simulink library "SG_library"  (R2020a)
settings: Solver=VariableStepAuto  StartTime=0.0  StopTime=10.0  RelTol=1e-3
undefined symbols (not defined in the file): a, b, c, IO334, IO334_IO_FPGA, IO334_IO_src, IO334_SOS_FPGA, IO334_SOS_src, IO397, IO397_IO_FPGA, IO397_IO_src, IO397_SOS_FPGA, IO397_SOS_src
libraries: speedgoatlib_hdlCoder_IO3xx x35, $bdroot x20, xpcutilitieslib x8, hdlsllib x5, simulink x4, simulink_extras x1
(part 1 of 2)
settings Model: Creator=mavolery  LastModifiedBy=mavolery
settings SFSimCC: CustomCodeUndefinedFunction=UseInterfaceOnly

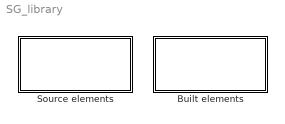
== system SG_library ==
  Built elements : Subsystem
  Source elements : Subsystem

== system SG_library/Built elements ==
  IO334_IO : Subsystem  mask(IO334 IO){ts=20e-6, OutputRange=Auto (same as ADC)}
      mask prompts: ts "Sampling time"; OutputRange "DAC Voltage Range:"
      mask help: Links the 16 first physical analog inputs/outputs to the CPU part of the speedgoat.
      mask TypeOptions OutputRange: IO334_IO_FPGA/OutputRange
      mask DialogControl AnalogOutput Prompt: Analog Output
  IO334_SOS : Subsystem  mask(IO334_SOS){sos1=[0 0 0 1 0 0;0 0 0 1 0 0;0 0 0 1 0 0;0 0 0 1 0 0], sos2=[0 0 0 1 0 0;0 0 0 1 0 0;0 0 0 1 0 0;0 0 0 1 0 0], limit_ctrl=10, ts=20e-6, os=1}
      mask prompts: sos1 "SOS matrix AI1 -> AO1"; sos2 "SOS matrix AI2 -> AO1"; limit_ctrl "Control output limit [V]"; ts "Sampling time (ADC)"; os "Oversampling (f_adc/f_cpu)"
      mask help: Implements a discrete fixed-point filter by second order sections cascade. SOS matrices are given by tf2sos or zp2sos.
  IO397_IO : Subsystem  mask(IO397 IO){ts=50e-6, range1=+-5 V, range2=+-5.12 V, range3=+-10 V, range4=+-10.24 V, span=+-10 V}
      mask prompts: ts "Sampling time:"; range1 "Range ADC Channel 1"; range2 "Range ADC Channel 2"; range3 "Range ADC Channel 3"; range4 "Range ADC Channel 4"; span "DAC Voltage Span:"
      mask help: Links the four first physical analog inputs/outputs to the CPU part of the speedgoat.
      mask TypeOptions range1: IO397_IO_FPGA/range1
      mask TypeOptions range2: IO397_IO_FPGA/range2
      mask TypeOptions range3: IO397_IO_FPGA/range3
      mask TypeOptions range4: IO397_IO_FPGA/range4
      mask TypeOptions span: IO397_IO_FPGA/span
      mask DialogControl AnalogInput Prompt: Analog Inputs
      mask DialogControl AnalogOutput Prompt: Analog Output
  IO397_SOS : Subsystem  mask(IO397_SOS){sos1=[1 0 0 1 0 0;1 0 0 1 0 0;1 0 0 1 0 0;1 0 0 1 0 0], sos2=[0 0 0 1 0 0;0 0 0 1 0 0;0 0 0 1 0 0;0 0 0 1 0 0], limit_ctrl=10, ts=50e-6, os=1, range1=+-10 V, range2=+-10 V, range3=+-10 V, range4=+-10 V, span=+-10 V}
      mask prompts: sos1 "SOS matrix AI1 -> AO1"; sos2 "SOS matrix AI2 -> AO1"; limit_ctrl "Control output limit [V]"; ts "Sampling time (ADC)"; os "Oversampling (f_adc/f_cpu)"; range1 "Range ADC Channel 1"; range2 "Range ADC Channel 2"; range3 "Range ADC Channel 3"; range4 "Range ADC Channel 4"; span "DAC Voltage Span:"
      mask help: Implements a discrete fixed-point filter by second order sections cascade. SOS matrices are given by tf2sos or zp2sos.
      mask init:
      | assert(all(range1 ~= [1 4 5]), 'ADC1 range must be symetric');
      | assert(all(range2 ~= [1 4 5]), 'ADC2 range must be symetric');
      | assert(all(span ~= [1 2]), 'DAC span must be symetric');
      mask TypeOptions range1: IO397_SOS_FPGA/range1
      mask TypeOptions range2: IO397_SOS_FPGA/range2
      mask TypeOptions range3: IO397_SOS_FPGA/range3
      mask TypeOptions range4: IO397_SOS_FPGA/range4
      mask TypeOptions span: IO397_SOS_FPGA/span
      mask DialogControl AnalogInput Prompt: Analog Inputs
      mask DialogControl AnalogOutput Prompt: Analog Output
  private : Subsystem

== system SG_library/Source elements ==
  ADC trigger : Subsystem  mask(AI trigger){}
      mask help: Creates a boolean pulse every given cylces. It can be use for ADC acquisition
  Discrete SOS section DFII serial : Subsystem  mask(Discrete fixed-point SOS section){idx=1}
      mask prompts: idx "Index"
      mask help:
      | This is a fixed-point implementation of a biquad filter. Specify the sos [N/2, 6] matrix e.g. given by tf2sos or zpk2sos functions. The first denominator coefficient must always be equal to 1. Index (1 - N/2) parameter specifies which section of the filter is implemented.
      |
      | This is the same implementation as in LabView VI "Discrete Transfer Function Direct.vi" or order 2. It has same fixed-point implementation too.
  Discrete SOS serial : Subsystem  mask(Discrete fixed-point second order sections filter){}
      mask help: This is a SOS implemetation of order 8 (4 sections). Specify the sos [n/2, 6] matrix e.g. given by tf2sos function. The first denominator coefficient must always be equal to 1.
  IO334 DAC double2fi : Subsystem  mask(DAC double2fi){span=1}
      mask help:
      | Converts the double signal to the fi(1,16,15) value for feeding the FPGA
      | Span is defined as follows:
      | 1 -> 0V - 5V
      | 2 -> 0V - 10V
      | 3 -> -5V - 5V
      | 4 -> -10V - 10V
  IO397 ADC fi2double : Subsystem  mask(ADC fi2double){range=1}
      mask help:
      | Converts the fi(1,16,15) signal from the FPGA to a double value
      | Range is defined as follows:
      | 1 -> 0V - 5.12V
      | 2 -> 0V - 10V (acts as -5V - 5V on IO397)
      | 3 -> 0V - 10.24V (acts as -5.12V - 5.12V on IO397)
      | 4 -> -5V - 5V (acts as 0V - 10V on IO397)
      | 5 -> -5.12V - 5.12V (acts as 0V - 10.24V on IO397)
      | 6 -> -10V - 10V
      | 7 -> -10.24V - 10.24V
  IO397 DAC double2fi : Subsystem  mask(DAC double2fi){span=1}
      mask help:
      | Converts the double signal to the fi(1,16,15) value for feeding the FPGA
      | Span is defined as follows:
      | 1 -> 0V - 5V
      | 2 -> 0V - 10V
      | 3 -> -5V - 5V
      | 4 -> -10V - 10V
  Random source : Subsystem  mask(Random source){mean=0, stdev=1, seed=0, SampleTime=0.0001}
      mask prompts: stdev "Standard deviation"; SampleTime "Sample time"
      mask help: Creates some random signal, limited in frequency at Fs/4
  Saturation : Subsystem  mask(Saturation){}
      mask help: Saturates the signal between -limit and limit.
  Triggered Pulse : Subsystem  mask(Triggered Pulse){}
      mask help: Generates a single pulse of N samples length

== system SG_library/Built elements/IO334_IO ==
  note: ADC range is not tuneable
  AO : Inport
  Data Type Conversion3 : DataTypeConversion  OutDataTypeStr=double
  Gain4 : Gain  Gain=20
  Ground : Ground
  IO334 DAC double2fi1 : $bdroot/Source elements/IO334 DAC double2fi  span=OutputRange
  IO334_IO_FPGA : $bdroot/Built elements/private/IO334_IO_FPGA  module_id=1  slot=-1  ts=-1  OutputRange=Auto (same as ADC)  FpgaFreq=100
  Mux : Mux  Inputs=26
  Rate Transition : RateTransition  OutPortSampleTime=ts
  Terminator : Terminator
  AI : Outport  VectorParamsAs1DForOutWhenUnconnected=off
  wires:
  AO/1 -> Rate Transition/1
  Data Type Conversion3/1 -> Gain4/1
  Gain4/1 -> AI/1
  IO334_IO_FPGA/27 -> Data Type Conversion3/1
  Rate Transition/1 -> IO334 DAC double2fi1/1
  IO334 DAC double2fi1/1 -> IO334_IO_FPGA/25
  Ground/1 -> IO334_IO_FPGA/1, IO334_IO_FPGA/2, IO334_IO_FPGA/3, IO334_IO_FPGA/4, IO334_IO_FPGA/5, IO334_IO_FPGA/6, IO334_IO_FPGA/7, IO334_IO_FPGA/8, IO334_IO_FPGA/9, IO334_IO_FPGA/10, IO334_IO_FPGA/11, IO334_IO_FPGA/12, IO334_IO_FPGA/13, IO334_IO_FPGA/14, IO334_IO_FPGA/15, IO334_IO_FPGA/16, IO334_IO_FPGA/17, IO334_IO_FPGA/18, IO334_IO_FPGA/19, IO334_IO_FPGA/20, IO334_IO_FPGA/21, IO334_IO_FPGA/22, IO334_IO_FPGA/23, IO334_IO_FPGA/24
  IO334_IO_FPGA/1 -> Mux/1
  IO334_IO_FPGA/2 -> Mux/2
  IO334_IO_FPGA/3 -> Mux/3
  IO334_IO_FPGA/4 -> Mux/4
  IO334_IO_FPGA/5 -> Mux/5
  IO334_IO_FPGA/6 -> Mux/6
  IO334_IO_FPGA/7 -> Mux/7
  IO334_IO_FPGA/8 -> Mux/8
  IO334_IO_FPGA/9 -> Mux/9
  IO334_IO_FPGA/10 -> Mux/10
  IO334_IO_FPGA/11 -> Mux/11
  IO334_IO_FPGA/12 -> Mux/12
  IO334_IO_FPGA/13 -> Mux/13
  IO334_IO_FPGA/14 -> Mux/14
  IO334_IO_FPGA/15 -> Mux/15
  IO334_IO_FPGA/16 -> Mux/16
  IO334_IO_FPGA/17 -> Mux/17
  IO334_IO_FPGA/18 -> Mux/18
  IO334_IO_FPGA/19 -> Mux/19
  IO334_IO_FPGA/20 -> Mux/20
  IO334_IO_FPGA/21 -> Mux/21
  IO334_IO_FPGA/22 -> Mux/22
  IO334_IO_FPGA/23 -> Mux/23
  IO334_IO_FPGA/24 -> Mux/24
  IO334_IO_FPGA/25 -> Mux/25
  IO334_IO_FPGA/26 -> Mux/26
  Mux/1 -> Terminator/1

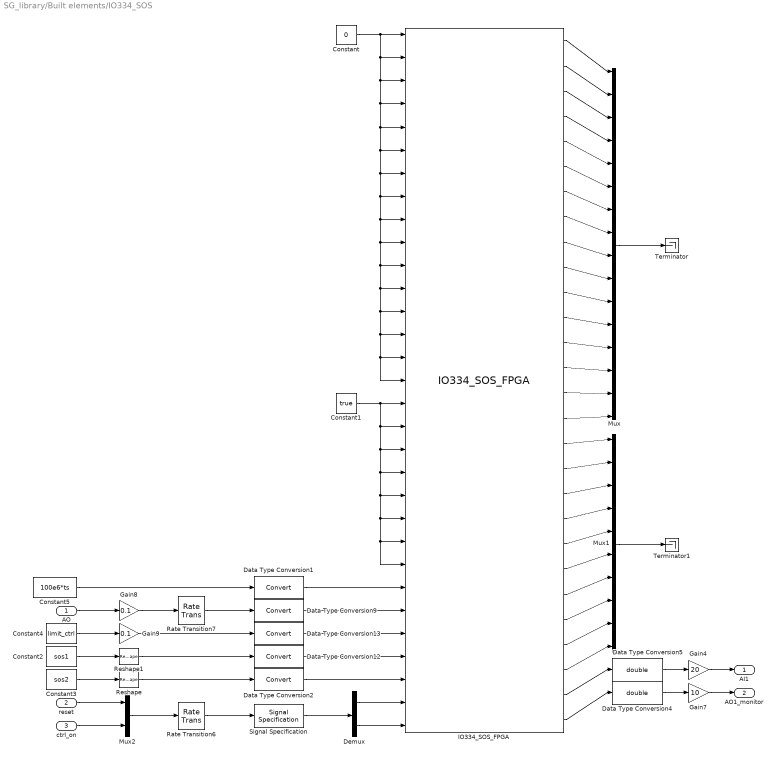
== system SG_library/Built elements/IO334_SOS ==
  AO : Inport
  reset : Inport  Port=2
  ctrl_on : Inport  Port=3
  Constant : Constant  Value=0  OutDataTypeStr=Inherit: Inherit via back propagation  SampleTime=-1
  Constant1 : Constant  Value=true  OutDataTypeStr=Inherit: Inherit via back propagation  SampleTime=-1
  Constant2 : Constant  Value=sos1  SampleTime=-1
  Constant3 : Constant  Value=sos2  SampleTime=-1
  Constant4 : Constant  Value=limit_ctrl  SampleTime=-1
  Constant5 : Constant  Value=100e6*ts  SampleTime=-1
  Data Type Conversion{1..2,9,12} (4 alike) : DataTypeConversion  RndMeth=Simplest
  Data Type Conversion13 : DataTypeConversion  RndMeth=Simplest  SaturateOnIntegerOverflow=on
  Data Type Conversion4 : DataTypeConversion  OutDataTypeStr=double
  Data Type Conversion5 : DataTypeConversion  OutDataTypeStr=double
  Demux : Demux  Outputs=2
  Gain4 : Gain  Gain=20
  Gain7 : Gain  Gain=10
  Gain8 : Gain  Gain=0.1
  Gain9 : Gain  Gain=0.1
  IO334_SOS_FPGA : $bdroot/Built elements/private/IO334_SOS_FPGA  module_id=1  slot=-1  ts=-1  OutputRange=Auto (same as ADC)  FpgaFreq=100
  Mux : Mux  Inputs=16
  Mux1 : Mux  Inputs=10
  Mux2 : Mux  Inputs=2
  Rate Transition6 : RateTransition
  Rate Transition7 : RateTransition  OutPortSampleTime=ts*os
  Reshape : Reshape
  Reshape1 : Reshape
  Signal Specification : SignalSpecification  OutDataTypeStr=boolean
  Terminator : Terminator
  Terminator1 : Terminator
  AI1 : Outport  VectorParamsAs1DForOutWhenUnconnected=off
  AO1_monitor : Outport  Port=2  VectorParamsAs1DForOutWhenUnconnected=off
  wires:
  Data Type Conversion5/1 -> Gain4/1
  Rate Transition6/1 -> Signal Specification/1
  Data Type Conversion4/1 -> Gain7/1
  Gain4/1 -> AI1/1
  Gain7/1 -> AO1_monitor/1
  Constant4/1 -> Gain9/1
  Gain9/1 -> Data Type Conversion13/1
  Signal Specification/1 -> Demux/1
  Constant2/1 -> Reshape1/1
  Constant3/1 -> Reshape/1
  Rate Transition7/1 -> Data Type Conversion9/1
  Gain8/1 -> Rate Transition7/1
  AO/1 -> Gain8/1
  Constant5/1 -> Data Type Conversion1/1
  Data Type Conversion1/1 -> IO334_SOS_FPGA/25
  Data Type Conversion9/1 -> IO334_SOS_FPGA/26
  Data Type Conversion13/1 -> IO334_SOS_FPGA/27
  Demux/2 -> IO334_SOS_FPGA/31
  Demux/1 -> IO334_SOS_FPGA/30
  Mux2/1 -> Rate Transition6/1
  ctrl_on/1 -> Mux2/2
  reset/1 -> Mux2/1
  Constant1/1 -> IO334_SOS_FPGA/17, IO334_SOS_FPGA/18, IO334_SOS_FPGA/19, IO334_SOS_FPGA/20, IO334_SOS_FPGA/21, IO334_SOS_FPGA/22, IO334_SOS_FPGA/23, IO334_SOS_FPGA/24
  Constant/1 -> IO334_SOS_FPGA/1, IO334_SOS_FPGA/2, IO334_SOS_FPGA/3, IO334_SOS_FPGA/4, IO334_SOS_FPGA/5, IO334_SOS_FPGA/6, IO334_SOS_FPGA/7, IO334_SOS_FPGA/8, IO334_SOS_FPGA/9, IO334_SOS_FPGA/10, IO334_SOS_FPGA/11, IO334_SOS_FPGA/12, IO334_SOS_FPGA/13, IO334_SOS_FPGA/14, IO334_SOS_FPGA/15, IO334_SOS_FPGA/16
  IO334_SOS_FPGA/1 -> Mux/1
  IO334_SOS_FPGA/2 -> Mux/2
  IO334_SOS_FPGA/3 -> Mux/3
  IO334_SOS_FPGA/4 -> Mux/4
  IO334_SOS_FPGA/5 -> Mux/5
  IO334_SOS_FPGA/6 -> Mux/6
  IO334_SOS_FPGA/7 -> Mux/7
  IO334_SOS_FPGA/8 -> Mux/8
  IO334_SOS_FPGA/9 -> Mux/9
  IO334_SOS_FPGA/10 -> Mux/10
  IO334_SOS_FPGA/11 -> Mux/11
  IO334_SOS_FPGA/12 -> Mux/12
  IO334_SOS_FPGA/13 -> Mux/13
  IO334_SOS_FPGA/14 -> Mux/14
  IO334_SOS_FPGA/15 -> Mux/15
  IO334_SOS_FPGA/16 -> Mux/16
  Mux/1 -> Terminator/1
  IO334_SOS_FPGA/17 -> Mux1/1
  IO334_SOS_FPGA/18 -> Mux1/2
  IO334_SOS_FPGA/19 -> Mux1/3
  IO334_SOS_FPGA/20 -> Mux1/4
  IO334_SOS_FPGA/21 -> Mux1/5
  IO334_SOS_FPGA/22 -> Mux1/6
  IO334_SOS_FPGA/23 -> Mux1/7
  IO334_SOS_FPGA/24 -> Mux1/8
  IO334_SOS_FPGA/25 -> Mux1/9
  IO334_SOS_FPGA/26 -> Mux1/10
  Mux1/1 -> Terminator1/1
  IO334_SOS_FPGA/28 -> Data Type Conversion4/1
  IO334_SOS_FPGA/27 -> Data Type Conversion5/1
  Data Type Conversion2/1 -> IO334_SOS_FPGA/29
  Data Type Conversion12/1 -> IO334_SOS_FPGA/28
  Reshape1/1 -> Data Type Conversion12/1
  Reshape/1 -> Data Type Conversion2/1

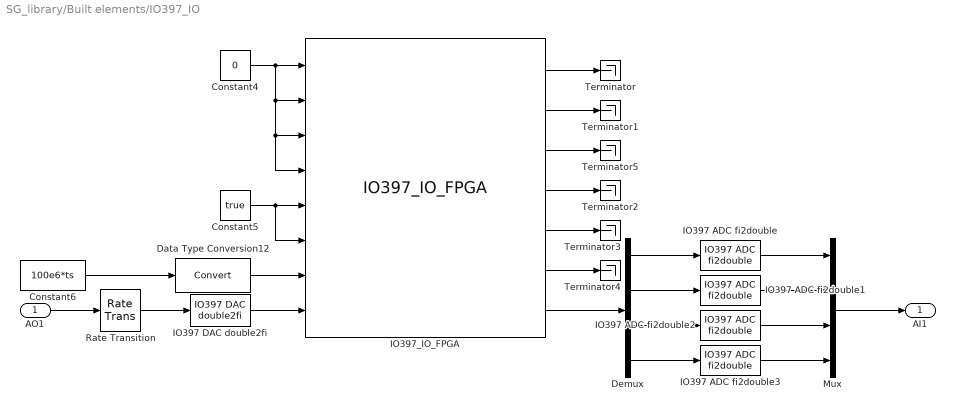
== system SG_library/Built elements/IO397_IO ==
  AO1 : Inport
  Constant4 : Constant  Value=0  OutDataTypeStr=fixdt(1,16,8)  SampleTime=-1
  Constant5 : Constant  Value=true  SampleTime=-1
  Constant6 : Constant  Value=100e6*ts  SampleTime=-1
  Data Type Conversion12 : DataTypeConversion  SaturateOnIntegerOverflow=on
  Demux : Demux
  IO397 ADC fi2double : $bdroot/Source elements/IO397 ADC fi2double  range=range1
  IO397 ADC fi2double1 : $bdroot/Source elements/IO397 ADC fi2double  range=range2
  IO397 ADC fi2double2 : $bdroot/Source elements/IO397 ADC fi2double  range=range3
  IO397 ADC fi2double3 : $bdroot/Source elements/IO397 ADC fi2double  range=range4
  IO397 DAC double2fi : $bdroot/Source elements/IO397 DAC double2fi  span=span
  IO397_IO_FPGA : $bdroot/Built elements/private/IO397_IO_FPGA  module_id=1  slot=-1  ts=-1  range1=+-5 V  range2=+-5.12 V  range3=+-10 V  range4=+-10.24 V  span=+-10 V  FpgaFreq=100
  Mux : Mux
  Rate Transition : RateTransition  OutPortSampleTime=ts
  Terminator{,1..5} (6 alike) : Terminator
  AI1 : Outport  VectorParamsAs1DForOutWhenUnconnected=off
  wires:
  Mux/1 -> AI1/1
  AO1/1 -> Rate Transition/1
  IO397_IO_FPGA/1 -> Terminator/1
  IO397_IO_FPGA/2 -> Terminator1/1
  IO397_IO_FPGA/4 -> Terminator2/1
  IO397_IO_FPGA/5 -> Terminator3/1
  IO397_IO_FPGA/6 -> Terminator4/1
  Constant4/1 -> IO397_IO_FPGA/1, IO397_IO_FPGA/4, IO397_IO_FPGA/3, IO397_IO_FPGA/2
  Constant5/1 -> IO397_IO_FPGA/6, IO397_IO_FPGA/5
  IO397_IO_FPGA/3 -> Terminator5/1
  Constant6/1 -> Data Type Conversion12/1
  Data Type Conversion12/1 -> IO397_IO_FPGA/7
  Rate Transition/1 -> IO397 DAC double2fi/1
  IO397 DAC double2fi/1 -> IO397_IO_FPGA/8
  IO397_IO_FPGA/7 -> Demux/1
  Demux/1 -> IO397 ADC fi2double/1
  Demux/2 -> IO397 ADC fi2double1/1
  Demux/3 -> IO397 ADC fi2double2/1
  Demux/4 -> IO397 ADC fi2double3/1
  IO397 ADC fi2double1/1 -> Mux/2
  IO397 ADC fi2double/1 -> Mux/1
  IO397 ADC fi2double2/1 -> Mux/3
  IO397 ADC fi2double3/1 -> Mux/4

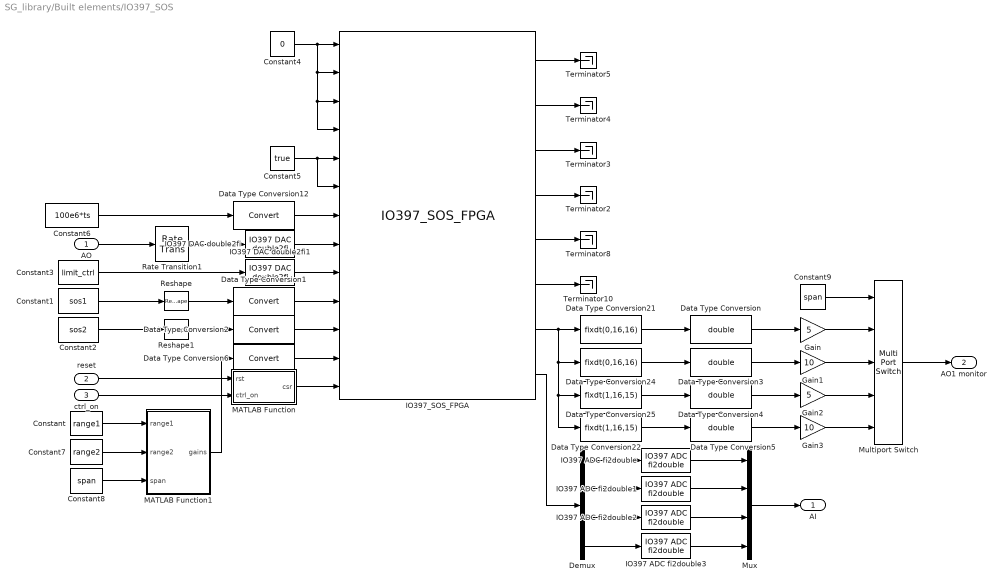
== system SG_library/Built elements/IO397_SOS ==
  AO : Inport
  reset : Inport  Port=2
  ctrl_on : Inport  Port=3
  Constant : Constant  Value=range1  SampleTime=-1
  Constant1 : Constant  Value=sos1  SampleTime=-1
  Constant2 : Constant  Value=sos2  SampleTime=-1
  Constant3 : Constant  Value=limit_ctrl  SampleTime=-1
  Constant4 : Constant  Value=0  OutDataTypeStr=fixdt(1,16,15)  SampleTime=-1
  Constant5 : Constant  Value=true  SampleTime=-1
  Constant6 : Constant  Value=100e6*ts  SampleTime=-1
  Constant7 : Constant  Value=range2  SampleTime=-1
  Constant8 : Constant  Value=span  SampleTime=-1
  Constant9 : Constant  Value=span  SampleTime=-1
  Data Type Conversion{,3..5} (4 alike) : DataTypeConversion  OutDataTypeStr=double
  Data Type Conversion{1..2,6,12} (4 alike) : DataTypeConversion  SaturateOnIntegerOverflow=on
  Data Type Conversion21 : DataTypeConversion  OutDataTypeStr=fixdt(0,16,16)  ConvertRealWorld=Stored Integer (SI)
  Data Type Conversion22 : DataTypeConversion  OutDataTypeStr=fixdt(1,16,15)  ConvertRealWorld=Stored Integer (SI)
  Data Type Conversion24 : DataTypeConversion  OutDataTypeStr=fixdt(0,16,16)  ConvertRealWorld=Stored Integer (SI)
  Data Type Conversion25 : DataTypeConversion  OutDataTypeStr=fixdt(1,16,15)  ConvertRealWorld=Stored Integer (SI)
  Demux : Demux
  Gain : Gain  Gain=5
  Gain1 : Gain  Gain=10
  Gain2 : Gain  Gain=5
  Gain3 : Gain  Gain=10
  IO397 ADC fi2double : $bdroot/Source elements/IO397 ADC fi2double  range=range1
  IO397 ADC fi2double1 : $bdroot/Source elements/IO397 ADC fi2double  range=range2
  IO397 ADC fi2double2 : $bdroot/Source elements/IO397 ADC fi2double  range=range3
  IO397 ADC fi2double3 : $bdroot/Source elements/IO397 ADC fi2double  range=range4
  IO397 DAC double2fi : $bdroot/Source elements/IO397 DAC double2fi  span=span
  IO397 DAC double2fi1 : $bdroot/Source elements/IO397 DAC double2fi  span=span
  IO397_SOS_FPGA : $bdroot/Built elements/private/IO397_SOS_FPGA  module_id=1  slot=-1  ts=-1  range1=+-10 V  range2=+-10 V  range3=+-10 V  range4=+-10 V  span=+-10 V  FpgaFreq=100
  MATLAB Function : MATLAB Function  TreatAsAtomicUnit=on
  MATLAB Function1 : MATLAB Function  TreatAsAtomicUnit=on
  Multiport Switch : MultiPortSwitch  Inputs=4
  Mux : Mux
  Rate Transition1 : RateTransition  OutPortSampleTime=ts*os
  Reshape : Reshape
  Reshape1 : Reshape
  Terminator{2..5,8,10} (6 alike) : Terminator
  AI : Outport  VectorParamsAs1DForOutWhenUnconnected=off
  AO1 monitor : Outport  Port=2  VectorParamsAs1DForOutWhenUnconnected=off
  wires:
  IO397_SOS_FPGA/2 -> Terminator4/1
  IO397_SOS_FPGA/6 -> Terminator10/1
  IO397_SOS_FPGA/5 -> Terminator8/1
  IO397_SOS_FPGA/4 -> Terminator2/1
  IO397_SOS_FPGA/3 -> Terminator3/1
  IO397_SOS_FPGA/1 -> Terminator5/1
  Data Type Conversion12/1 -> IO397_SOS_FPGA/7
  Constant6/1 -> Data Type Conversion12/1
  Constant4/1 -> IO397_SOS_FPGA/1, IO397_SOS_FPGA/2, IO397_SOS_FPGA/3, IO397_SOS_FPGA/4
  Constant5/1 -> IO397_SOS_FPGA/5, IO397_SOS_FPGA/6
  Reshape/1 -> Data Type Conversion1/1
  Constant1/1 -> Reshape/1
  Constant2/1 -> Reshape1/1
  Reshape1/1 -> Data Type Conversion2/1
  Data Type Conversion2/1 -> IO397_SOS_FPGA/11
  Data Type Conversion1/1 -> IO397_SOS_FPGA/10
  Rate Transition1/1 -> IO397 DAC double2fi/1
  AO/1 -> Rate Transition1/1
  IO397 DAC double2fi1/1 -> IO397_SOS_FPGA/9
  IO397 DAC double2fi/1 -> IO397_SOS_FPGA/8
  Constant3/1 -> IO397 DAC double2fi1/1
  MATLAB Function/1(csr) -> IO397_SOS_FPGA/13
  reset/1 -> MATLAB Function/1(rst)
  ctrl_on/1 -> MATLAB Function/2(ctrl_on)
  MATLAB Function1/1(gains) -> Data Type Conversion6/1
  Constant/1 -> MATLAB Function1/1(range1)
  Constant7/1 -> MATLAB Function1/2(range2)
  Constant8/1 -> MATLAB Function1/3(span)
  Data Type Conversion21/1 -> Data Type Conversion/1
  Data Type Conversion24/1 -> Data Type Conversion3/1
  Data Type Conversion25/1 -> Data Type Conversion4/1
  Data Type Conversion22/1 -> Data Type Conversion5/1
  IO397_SOS_FPGA/7 -> Data Type Conversion21/1, Data Type Conversion24/1, Data Type Conversion25/1, Data Type Conversion22/1
  Data Type Conversion/1 -> Gain/1
  Data Type Conversion3/1 -> Gain1/1
  Data Type Conversion4/1 -> Gain2/1
  Data Type Conversion5/1 -> Gain3/1
  Gain/1 -> Multiport Switch/2
  Gain1/1 -> Multiport Switch/3
  Gain2/1 -> Multiport Switch/4
  Gain3/1 -> Multiport Switch/5
  Multiport Switch/1 -> AO1 monitor/1
  Constant9/1 -> Multiport Switch/1
  IO397 ADC fi2double2/1 -> Mux/3
  IO397 ADC fi2double/1 -> Mux/1
  IO397 ADC fi2double3/1 -> Mux/4
  Demux/3 -> IO397 ADC fi2double2/1
  IO397_SOS_FPGA/8 -> Demux/1
  Demux/2 -> IO397 ADC fi2double1/1
  IO397 ADC fi2double1/1 -> Mux/2
  Demux/4 -> IO397 ADC fi2double3/1
  Mux/1 -> AI/1
  Demux/1 -> IO397 ADC fi2double/1
  Data Type Conversion6/1 -> IO397_SOS_FPGA/12

== system SG_library/Built elements/private ==
  IO334_IO_FPGA : Subsystem  mask(Speedgoat IO334-325k Interface Block){module_id=1, slot=-1, ts=-1, OutputRange=Auto (same as ADC), FpgaFreq=100}
      mask prompts: module_id "FPGA Module Identifier:"; slot "PCI slot (-1: autosearch):"; ts "Sample time:"; OutputRange "DAC Voltage Range:"; FpgaFreq "FPGA Frequency [MHz]"
      mask help: Simulink Real-Time Interface Block for Speedgoat IO334-325k.
      mask init:
      | mfpgaparameters;
      mask Help: eval('speedgoatdoc_hdlc')
      mask TypeOptions OutputRange: IO334 DAC Setup/OutputRange
      mask DialogControl AnalogOutput Prompt: Analog Output
      mask Display:
      | SetupBlkPath = find_system(gcb, 'LookUnderMasks', 'all', 'FollowLinks', 'on', 'regexp', 'on', 'Name', 'IO3(\d|x){2}\s+Setup' );
      | SetupBlkPath = SetupBlkPath{1};
      | TS = get_param(SetupBlkPath,'timestamp_mcs');
      | disp(sprintf('Speedgoat IO334-325k\nFPGA I/O Module\n\nTimestamp\n%s\n\nReference Design\nVersion 1.4\n\nMatlab R2020a\n\nPCIe Link Width: X4\nRear Plugin: None\nAurora Mode: None\nAurora Byteswap: true\n', TS))
  IO334_SOS_FPGA : Subsystem  mask(Speedgoat IO334-325k Interface Block){module_id=1, slot=-1, ts=-1, OutputRange=Auto (same as ADC), FpgaFreq=100}
      mask prompts: module_id "FPGA Module Identifier:"; slot "PCI slot (-1: autosearch):"; ts "Sample time:"; OutputRange "DAC Voltage Range:"; FpgaFreq "FPGA Frequency [MHz]"
      mask help: Simulink Real-Time Interface Block for Speedgoat IO334-325k.
      mask init:
      | mfpgaparameters;
      mask Help: eval('speedgoatdoc_hdlc')
      mask TypeOptions OutputRange: IO334 DAC Setup/OutputRange
      mask DialogControl AnalogOutput Prompt: Analog Output
      mask Display:
      | SetupBlkPath = find_system(gcb, 'LookUnderMasks', 'all', 'FollowLinks', 'on', 'regexp', 'on', 'Name', 'IO3(\d|x){2}\s+Setup' );
      | SetupBlkPath = SetupBlkPath{1};
      | TS = get_param(SetupBlkPath,'timestamp_mcs');
      | disp(sprintf('Speedgoat IO334-325k\nFPGA I/O Module\n\nTimestamp\n%s\n\nReference Design\nVersion 1.4\n\nMatlab R2020a\n\nPCIe Link Width: X4\nRear Plugin: None\nAurora Mode: None\nAurora Byteswap: true\n', TS))
  IO397_IO_FPGA : Subsystem  mask(Speedgoat IO397-50k Interface Block){module_id=1, slot=-1, ts=-1, range1=+-10 V, range2=+-10 V, range3=+-10 V, range4=+-10 V, span=+-10 V, FpgaFreq=100}
      mask prompts: module_id "FPGA Module Identifier:"; slot "PCI slot (-1: autosearch):"; ts "Sample time:"; range1 "Range ADC Channel 1"; range2 "Range ADC Channel 2"; range3 "Range ADC Channel 3"; range4 "Range ADC Channel 4"; span "DAC Voltage Span:"; FpgaFreq "FPGA Frequency [MHz]"
      mask help: Simulink Real-Time Interface Block for Speedgoat IO397-50k.
      mask init:
      | mfpgaparameters;
      mask Help: eval('speedgoatdoc_hdlc')
      mask TypeOptions range1: IO397 ADC Setup/range1
      mask TypeOptions range2: IO397 ADC Setup/range2
      mask TypeOptions range3: IO397 ADC Setup/range3
      mask TypeOptions range4: IO397 ADC Setup/range4
      mask TypeOptions span: IO397 DAC Setup/span
      mask DialogControl AnalogInput Prompt: Analog Input
      mask DialogControl AnalogOutput Prompt: Analog Output
      mask Display:
      | SetupBlkPath = find_system(gcb, 'LookUnderMasks', 'all', 'FollowLinks', 'on', 'regexp', 'on', 'Name', 'IO3(\d|x){2}\s+Setup' );
      | SetupBlkPath = SetupBlkPath{1};
      | TS = get_param(SetupBlkPath,'timestamp_mcs');
      | disp(sprintf('Speedgoat IO397-50k\nFPGA I/O Module\n\nTimestamp\n%s\n\nReference Design\nVersion 1.4\n\nMatlab R2020a\n\nPCIe Link Width: X1\n', TS))
  IO397_SOS_FPGA : Subsystem  mask(Speedgoat IO397-50k Interface Block){module_id=1, slot=-1, ts=-1, range1=+-10 V, range2=+-10 V, range3=+-10 V, range4=+-10 V, span=+-10 V, FpgaFreq=100}
      mask prompts: module_id "FPGA Module Identifier:"; slot "PCI slot (-1: autosearch):"; ts "Sample time:"; range1 "Range ADC Channel 1"; range2 "Range ADC Channel 2"; range3 "Range ADC Channel 3"; range4 "Range ADC Channel 4"; span "DAC Voltage Span:"; FpgaFreq "FPGA Frequency [MHz]"
      mask help: Simulink Real-Time Interface Block for Speedgoat IO397-50k.
      mask init:
      | mfpgaparameters;
      mask Help: eval('speedgoatdoc_hdlc')
      mask TypeOptions range1: IO397 ADC Setup/range1
      mask TypeOptions range2: IO397 ADC Setup/range2
      mask TypeOptions range3: IO397 ADC Setup/range3
      mask TypeOptions range4: IO397 ADC Setup/range4
      mask TypeOptions span: IO397 DAC Setup/span
      mask DialogControl AnalogInput Prompt: Analog Input
      mask DialogControl AnalogOutput Prompt: Analog Output
      mask Display:
      | SetupBlkPath = find_system(gcb, 'LookUnderMasks', 'all', 'FollowLinks', 'on', 'regexp', 'on', 'Name', 'IO3(\d|x){2}\s+Setup' );
      | SetupBlkPath = SetupBlkPath{1};
      | TS = get_param(SetupBlkPath,'timestamp_mcs');
      | disp(sprintf('Speedgoat IO397-50k\nFPGA I/O Module\n\nTimestamp\n%s\n\nReference Design\nVersion 1.4\n\nMatlab R2020a\n\nPCIe Link Width: X1\n', TS))

== system SG_library/Source elements/ADC trigger ==
  ticks : Inport
  Decrement Stored Integer : simulink/Additional Math & Discrete/Additional Math: Increment - Decrement/Decrement Stored Integer
      settings: SourceProductBaseCode=SL
  HDL Counter3 : hdlsllib/Sources/HDL Counter  CountType=Free running  CountInit=uint32(0)  CountStep=uint32(1)  CountMax=25  CountFromType=Initial value  CountFrom=uint32(0)  CountResetPort=on  CountLoadPort=off  CountEnbPort=off  CountDirPort=off  CountDataType=Unsigned  CountWordLen=32  CountFracLen=0  CountSampTime=1
  Relational Operator1 : RelationalOperator  Operator=<=  OutDataTypeStr=boolean  RndMeth=Simplest
  trig : Outport  VectorParamsAs1DForOutWhenUnconnected=off
  wires:
  HDL Counter3/1 -> Relational Operator1/2
  Relational Operator1/1 -> HDL Counter3/1, trig/1
  ticks/1 -> Decrement Stored Integer/1
  Decrement Stored Integer/1 -> Relational Operator1/1

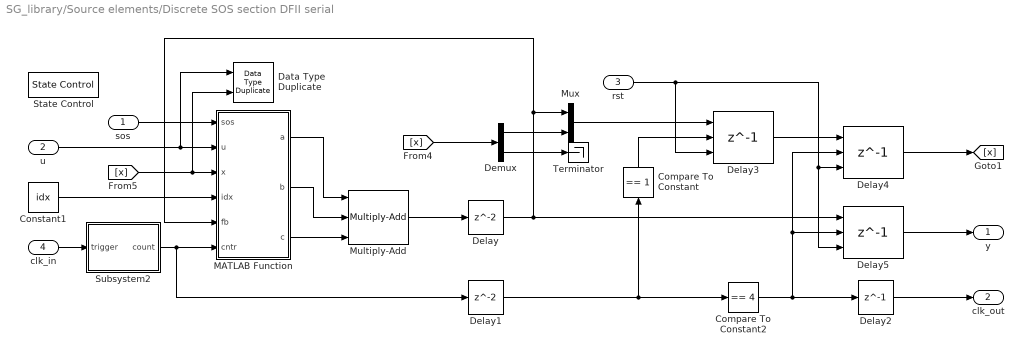
== system SG_library/Source elements/Discrete SOS section DFII serial ==
  sos : Inport
  u : Inport  Port=2
  rst : Inport  Port=3
  clk_in : Inport  Port=4
  Compare To Constant : simulink/Logic and Bit Operations/Compare To Constant  relop===  const=1  OutDataTypeStr=boolean
  Compare To Constant2 : simulink/Logic and Bit Operations/Compare To Constant  relop===  const=4  OutDataTypeStr=boolean
  Constant1 : Constant  Value=idx  OutDataTypeStr=uint8  SampleTime=-1
  Data Type Duplicate : DataTypeDuplicate
  Delay : Delay
  Delay1 : Delay
  Delay2 : Delay  DelayLength=1
  Delay3 : Delay  DelayLength=1  ExternalReset=Level hold  ShowEnablePort=on
      settings: InputPortMap=u0,e6,r5
  Delay4 : Delay  DelayLength=1  ExternalReset=Level hold  ShowEnablePort=on
      settings: InputPortMap=u0,e6,r5
  Delay5 : Delay  DelayLength=1  ExternalReset=Level hold  ShowEnablePort=on
      settings: InputPortMap=u0,e6,r5
  Demux : Demux  Outputs=2
  MATLAB Function : MATLAB Function  TreatAsAtomicUnit=on
  Multiply-Add : hdlsllib/HDL Operations/Multiply-Add  Function=c+(a.*b)  datatype=Inherit: Same as first input  RndMeth=Simplest  DoSatur=on  FMA=off
      settings: SourceProductBaseCode=SL
  Mux : Mux  Inputs=2
  State Control : StateControl  StateControl=Synchronous
  Subsystem2 : Subsystem
  Terminator : Terminator
  y : Outport  InitialOutput=0  VectorParamsAs1DForOutWhenUnconnected=off
  clk_out : Outport  Port=2
  wires:
  Delay5/1 -> y/1
  sos/1 -> MATLAB Function/1(sos)
  [x] -> Data Type Duplicate/2, MATLAB Function/3(x)
  Delay1/1 -> Compare To Constant2/1, Compare To Constant/1
  Constant1/1 -> MATLAB Function/4(idx)
  rst/1 -> Delay3/3, Delay5/3, Delay4/3
  Compare To Constant/1 -> Delay3/2
  Delay2/1 -> clk_out/1
  Delay3/1 -> Delay4/1
  Delay4/1 -> [x]
  u/1 -> Data Type Duplicate/1, MATLAB Function/2(u)
  Subsystem2/1(count) -> Delay1/1, MATLAB Function/6(cntr)
  clk_in/1 -> Subsystem2/1(trigger)
  Mux/1 -> Delay3/1
  [x] -> Demux/1
  Demux/2 -> Terminator/1
  Demux/1 -> Mux/2
  Multiply-Add/1 -> Delay/1
  MATLAB Function/3(c) -> Multiply-Add/3
  Delay/1 -> MATLAB Function/5(fb), Mux/1, Delay5/1
  Compare To Constant2/1 -> Delay2/1, Delay5/2, Delay4/2
  MATLAB Function/2(b) -> Multiply-Add/2
  MATLAB Function/1(a) -> Multiply-Add/1

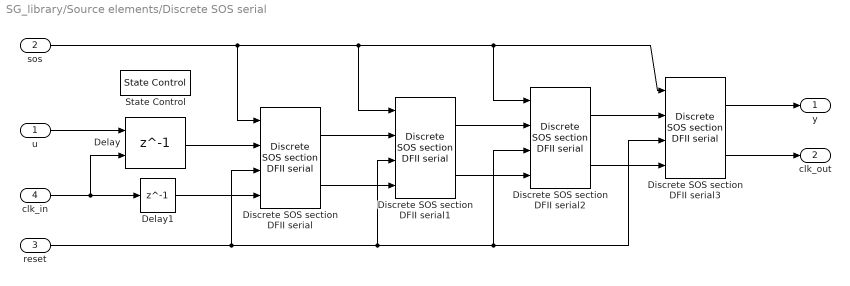
== system SG_library/Source elements/Discrete SOS serial ==
  u : Inport
  sos : Inport  Port=2
  reset : Inport  Port=3
  clk_in : Inport  Port=4
  Delay : Delay  DelayLength=1  ShowEnablePort=on
      settings: InputPortMap=u0,e6
  Delay1 : Delay  DelayLength=1
  Discrete SOS section DFII serial : $bdroot/Source elements/Discrete SOS section DFII serial  idx=1
  Discrete SOS section DFII serial1 : $bdroot/Source elements/Discrete SOS section DFII serial  idx=2
  Discrete SOS section DFII serial2 : $bdroot/Source elements/Discrete SOS section DFII serial  idx=3
  Discrete SOS section DFII serial3 : $bdroot/Source elements/Discrete SOS section DFII serial  idx=4
  State Control : StateControl  StateControl=Synchronous
  y : Outport  InitialOutput=0  VectorParamsAs1DForOutWhenUnconnected=off
  clk_out : Outport  Port=2
  wires:
  Delay/1 -> Discrete SOS section DFII serial/2
  sos/1 -> Discrete SOS section DFII serial/1, Discrete SOS section DFII serial1/1, Discrete SOS section DFII serial2/1, Discrete SOS section DFII serial3/1
  Discrete SOS section DFII serial2/1 -> Discrete SOS section DFII serial3/2
  Discrete SOS section DFII serial1/1 -> Discrete SOS section DFII serial2/2
  Discrete SOS section DFII serial/1 -> Discrete SOS section DFII serial1/2
  Discrete SOS section DFII serial/2 -> Discrete SOS section DFII serial1/4
  Discrete SOS section DFII serial1/2 -> Discrete SOS section DFII serial2/4
  Discrete SOS section DFII serial2/2 -> Discrete SOS section DFII serial3/4
  Discrete SOS section DFII serial3/2 -> clk_out/1
  Discrete SOS section DFII serial3/1 -> y/1
  clk_in/1 -> Delay1/1, Delay/2
  u/1 -> Delay/1
  Delay1/1 -> Discrete SOS section DFII serial/4
  reset/1 -> Discrete SOS section DFII serial/3, Discrete SOS section DFII serial1/3, Discrete SOS section DFII serial2/3, Discrete SOS section DFII serial3/3

== system SG_library/Source elements/IO334 DAC double2fi ==
  in : Inport
  Constant : Constant  Value=span  SampleTime=-1
  Data Type Conversion : DataTypeConversion  OutDataTypeStr=fixdt(1,16,15)  RndMeth=Convergent  SaturateOnIntegerOverflow=on
  Gain1 : Gain  Gain=0.1
  Gain2 : Gain  Gain=0.2
  Gain3 : Gain  Gain=0.4
  Multiport Switch : MultiPortSwitch  Inputs=4
  out : Outport
  wires:
  Gain3/1 -> Multiport Switch/5
  Gain2/1 -> Multiport Switch/4
  Multiport Switch/1 -> Data Type Conversion/1
  in/1 -> Gain1/1, Gain2/1, Gain3/1
  Gain1/1 -> Multiport Switch/2, Multiport Switch/3
  Data Type Conversion/1 -> out/1
  Constant/1 -> Multiport Switch/1

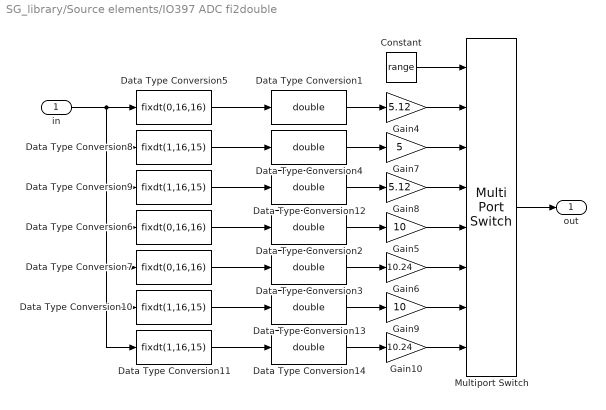
== system SG_library/Source elements/IO397 ADC fi2double ==
  in : Inport
  Constant : Constant  Value=range  SampleTime=-1
  Data Type Conversion{1..4,12..14} (7 alike) : DataTypeConversion  OutDataTypeStr=double  RndMeth=Convergent  SaturateOnIntegerOverflow=on
  Data Type Conversion{8..11} (4 alike) : DataTypeConversion  OutDataTypeStr=fixdt(1,16,15)  ConvertRealWorld=Stored Integer (SI)
  Data Type Conversion5 : DataTypeConversion  OutDataTypeStr=fixdt(0,16,16)  ConvertRealWorld=Stored Integer (SI)
  Data Type Conversion6 : DataTypeConversion  OutDataTypeStr=fixdt(0,16,16)  ConvertRealWorld=Stored Integer (SI)
  Data Type Conversion7 : DataTypeConversion  OutDataTypeStr=fixdt(0,16,16)  ConvertRealWorld=Stored Integer (SI)
  Gain10 : Gain  Gain=10.24
  Gain4 : Gain  Gain=5.12
  Gain5 : Gain  Gain=10
  Gain6 : Gain  Gain=10.24
  Gain7 : Gain  Gain=5
  Gain8 : Gain  Gain=5.12
  Gain9 : Gain  Gain=10
  Multiport Switch : MultiPortSwitch  Inputs=7
  out : Outport
  wires:
  Data Type Conversion8/1 -> Data Type Conversion4/1
  Data Type Conversion4/1 -> Gain7/1
  Gain7/1 -> Multiport Switch/3
  Gain8/1 -> Multiport Switch/4
  Data Type Conversion9/1 -> Data Type Conversion12/1
  Data Type Conversion12/1 -> Gain8/1
  Data Type Conversion6/1 -> Data Type Conversion2/1
  in/1 -> Data Type Conversion5/1, Data Type Conversion8/1, Data Type Conversion9/1, Data Type Conversion11/1, Data Type Conversion10/1, Data Type Conversion7/1, Data Type Conversion6/1
  Data Type Conversion7/1 -> Data Type Conversion3/1
  Data Type Conversion2/1 -> Gain5/1
  Data Type Conversion3/1 -> Gain6/1
  Gain5/1 -> Multiport Switch/5
  Gain6/1 -> Multiport Switch/6
  Gain9/1 -> Multiport Switch/7
  Multiport Switch/1 -> out/1
  Data Type Conversion10/1 -> Data Type Conversion13/1
  Data Type Conversion1/1 -> Gain4/1
  Data Type Conversion11/1 -> Data Type Conversion14/1
  Gain10/1 -> Multiport Switch/8
  Gain4/1 -> Multiport Switch/2
  Data Type Conversion13/1 -> Gain9/1
  Data Type Conversion14/1 -> Gain10/1
  Data Type Conversion5/1 -> Data Type Conversion1/1
  Constant/1 -> Multiport Switch/1

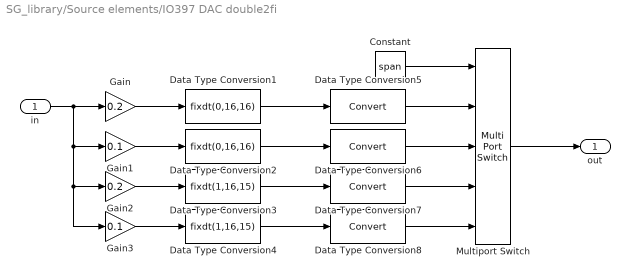
== system SG_library/Source elements/IO397 DAC double2fi ==
  in : Inport
  Constant : Constant  Value=span  SampleTime=-1
  Data Type Conversion1 : DataTypeConversion  OutDataTypeStr=fixdt(0,16,16)  RndMeth=Convergent  SaturateOnIntegerOverflow=on
  Data Type Conversion2 : DataTypeConversion  OutDataTypeStr=fixdt(0,16,16)  RndMeth=Convergent  SaturateOnIntegerOverflow=on
  Data Type Conversion3 : DataTypeConversion  OutDataTypeStr=fixdt(1,16,15)  RndMeth=Convergent  SaturateOnIntegerOverflow=on
  Data Type Conversion4 : DataTypeConversion  OutDataTypeStr=fixdt(1,16,15)  RndMeth=Convergent  SaturateOnIntegerOverflow=on
  Data Type Conversion{5..8} (4 alike) : DataTypeConversion  ConvertRealWorld=Stored Integer (SI)
  Gain : Gain  Gain=0.2
  Gain1 : Gain  Gain=0.1
  Gain2 : Gain  Gain=0.2
  Gain3 : Gain  Gain=0.1
  Multiport Switch : MultiPortSwitch  Inputs=4
  out : Outport
  wires:
  Data Type Conversion4/1 -> Data Type Conversion8/1
  Gain3/1 -> Data Type Conversion4/1
  Gain2/1 -> Data Type Conversion3/1
  Data Type Conversion5/1 -> Multiport Switch/2
  Gain/1 -> Data Type Conversion1/1
  Data Type Conversion1/1 -> Data Type Conversion5/1
  Data Type Conversion3/1 -> Data Type Conversion7/1
  Gain1/1 -> Data Type Conversion2/1
  Data Type Conversion2/1 -> Data Type Conversion6/1
  Data Type Conversion6/1 -> Multiport Switch/3
  Data Type Conversion8/1 -> Multiport Switch/5
  Data Type Conversion7/1 -> Multiport Switch/4
  in/1 -> Gain3/1, Gain2/1, Gain1/1, Gain/1
  Multiport Switch/1 -> out/1
  Constant/1 -> Multiport Switch/1

== system SG_library/Source elements/Random source ==
  Discrete Filter : DiscreteFilter  Numerator=[0.5 0.5]  Denominator=[1 0.1]  InputProcessing=Columns as channels (frame based)  FilterStructure=Direct form II transposed  a0EqualsOne=on
  Random Number : RandomNumber  Mean=mean  Variance=stdev^2  Seed=seed  SampleTime=SampleTime
  x : Outport  VectorParamsAs1DForOutWhenUnconnected=off
  wires:
  Random Number/1 -> Discrete Filter/1
  Discrete Filter/1 -> x/1

== system SG_library/Source elements/Saturation ==
  in : Inport
  limit : Inport  Port=2
  Relational Operator : RelationalOperator  Operator=<  OutDataTypeStr=boolean  RndMeth=Simplest
  Relational Operator1 : RelationalOperator  Operator=>  OutDataTypeStr=boolean  RndMeth=Simplest
  Switch : Switch  Criteria=u2 > Threshold
  Switch1 : Switch  Criteria=u2 > Threshold
  Unary Minus : UnaryMinus
  out : Outport
  wires:
  Relational Operator/1 -> Switch/2
  in/1 -> Switch/1, Relational Operator/1
  Switch1/1 -> out/1
  Relational Operator1/1 -> Switch1/2
  limit/1 -> Switch/3, Unary Minus/1, Relational Operator/2
  Switch/1 -> Relational Operator1/1, Switch1/1
  Unary Minus/1 -> Switch1/3, Relational Operator1/2

== system SG_library/Source elements/Triggered Pulse ==
  trigger : Inport
  reset : Inport  Port=2
  N : Inport  Port=3
  HDL Counter : hdlsllib/Sources/HDL Counter  CountType=Free running  CountInit=0  CountStep=1  CountMax=25  CountFromType=Initial value  CountFrom=0  CountResetPort=on  CountLoadPort=off  CountEnbPort=on  CountDirPort=off  CountDataType=Unsigned  CountWordLen=32  CountFracLen=0  CountSampTime=1
  OR : Logic  Operator=OR  AllPortsSameDT=off  OutDataTypeStr=boolean
  S-R Flip-Flop : simulink_extras/Flip Flops/S-R Flip-Flop  initial_condition=0
  Terminator : Terminator
  cntr full? : RelationalOperator  OutDataTypeStr=boolean  RndMeth=Simplest
  pulse : Outport  VectorParamsAs1DForOutWhenUnconnected=off
  wires:
  cntr full?/1 -> OR/2
  reset/1 -> OR/1
  OR/1 -> HDL Counter/1, S-R Flip-Flop/2
  S-R Flip-Flop/2 -> Terminator/1
  trigger/1 -> S-R Flip-Flop/1
  N/1 -> cntr full?/2
  S-R Flip-Flop/1 -> HDL Counter/2, pulse/1
  HDL Counter/1 -> cntr full?/1

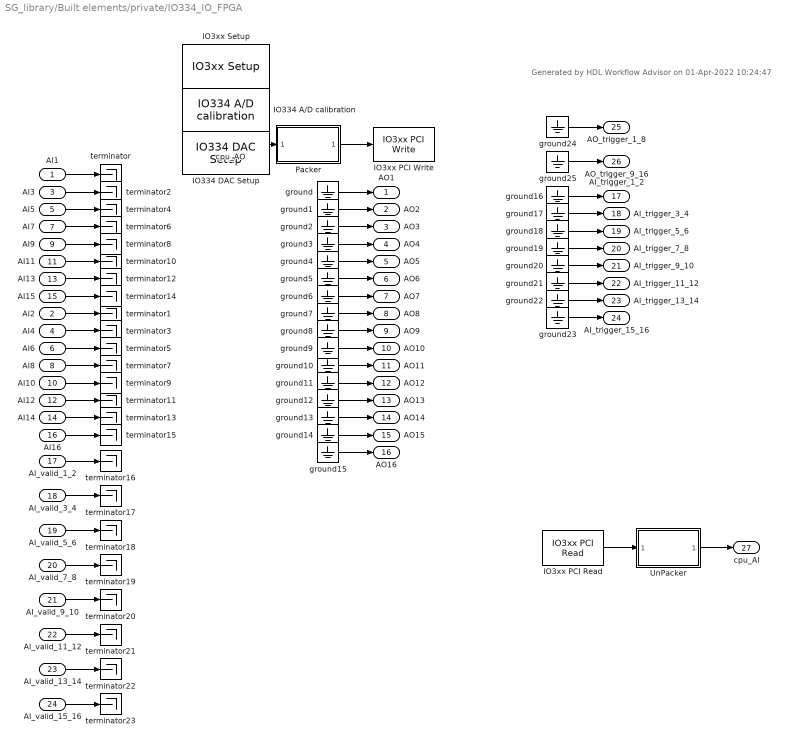
== system SG_library/Built elements/private/IO334_IO_FPGA ==
  note: Generated by HDL Workflow Advisor on 01-Apr-2022 10:24:47
  AI1 : Inport
  AI2 : Inport  Port=2
  AI3 : Inport  Port=3
  AI4 : Inport  Port=4
  AI5 : Inport  Port=5
  AI6 : Inport  Port=6
  AI7 : Inport  Port=7
  AI8 : Inport  Port=8
  AI9 : Inport  Port=9
  AI10 : Inport  Port=10
  AI11 : Inport  Port=11
  AI12 : Inport  Port=12
  AI13 : Inport  Port=13
  AI14 : Inport  Port=14
  AI15 : Inport  Port=15
  AI16 : Inport  Port=16
  AI_valid_1_2 : Inport  Port=17
  AI_valid_3_4 : Inport  Port=18
  AI_valid_5_6 : Inport  Port=19
  AI_valid_7_8 : Inport  Port=20
  AI_valid_9_10 : Inport  Port=21
  AI_valid_11_12 : Inport  Port=22
  AI_valid_13_14 : Inport  Port=23
  AI_valid_15_16 : Inport  Port=24
  cpu_AO : Inport  Port=25
  IO334 A/D calibration : speedgoatlib_hdlCoder_IO3xx/IO334 A//D calibration  module_id=module_id
  IO334 DAC Setup : speedgoatlib_hdlCoder_IO3xx/IO334 DAC Setup  module_id=module_id  OutputRange=Auto (same as ADC)
  IO3xx PCI Read : speedgoatlib_hdlCoder_IO3xx/IO3xx PCI Read  device_id=deviceIdx  module_id=module_id  board_type=IO3xx  port_name=cpu_AI  port_offset=hex2dec('140')  port_type=uint32  port_dim=8  strobe=hex2dec('160')  sample_time=ts
  IO3xx PCI Write : speedgoatlib_hdlCoder_IO3xx/IO3xx PCI Write  device_id=deviceIdx  module_id=module_id  board_type=IO3xx  port_name=cpu_AO  port_offset=hex2dec('100')  port_type=uint32  port_dim=8  strobe=hex2dec('120')  sample_time=ts
  IO3xx Setup : speedgoatlib_hdlCoder_IO3xx/IO3xx Setup  mdl_ss_name=IO334_IO_src/IO334_IO_FPGA  board_type=IO334-325k  fpga_sync_mode=on  reset_mode=on  device_id=deviceIdx  module_id=module_id  pci_slot=slot  fpga_mat_file=C:\Speedgoat\Build\IO334_IO\hdlsrc\IO334_IO_src\IO334_IO_FPGA.mat  timestamp_mcs=04/01/22 09:48:38  timestamp=2204010923  tsreg=hex2dec('8')  bsf_file=IO334_IO_FPGA_2204010923.mcs  mcs=0
  Packer : Subsystem
  UnPacker : Subsystem
  ground{,1..25} (26 alike) : Ground
  terminator{,1..23} (24 alike) : Terminator
  AO1 : Outport  VectorParamsAs1DForOutWhenUnconnected=off
  AO2 : Outport  Port=2  VectorParamsAs1DForOutWhenUnconnected=off
  AO3 : Outport  Port=3  VectorParamsAs1DForOutWhenUnconnected=off
  AO4 : Outport  Port=4  VectorParamsAs1DForOutWhenUnconnected=off
  AO5 : Outport  Port=5  VectorParamsAs1DForOutWhenUnconnected=off
  AO6 : Outport  Port=6  VectorParamsAs1DForOutWhenUnconnected=off
  AO7 : Outport  Port=7  VectorParamsAs1DForOutWhenUnconnected=off
  AO8 : Outport  Port=8  VectorParamsAs1DForOutWhenUnconnected=off
  AO9 : Outport  Port=9  VectorParamsAs1DForOutWhenUnconnected=off
  AO10 : Outport  Port=10  VectorParamsAs1DForOutWhenUnconnected=off
  AO11 : Outport  Port=11  VectorParamsAs1DForOutWhenUnconnected=off
  AO12 : Outport  Port=12  VectorParamsAs1DForOutWhenUnconnected=off
  AO13 : Outport  Port=13  VectorParamsAs1DForOutWhenUnconnected=off
  AO14 : Outport  Port=14  VectorParamsAs1DForOutWhenUnconnected=off
  AO15 : Outport  Port=15  VectorParamsAs1DForOutWhenUnconnected=off
  AO16 : Outport  Port=16  VectorParamsAs1DForOutWhenUnconnected=off
  AI_trigger_1_2 : Outport  Port=17  VectorParamsAs1DForOutWhenUnconnected=off
  AI_trigger_3_4 : Outport  Port=18  VectorParamsAs1DForOutWhenUnconnected=off
  AI_trigger_5_6 : Outport  Port=19  VectorParamsAs1DForOutWhenUnconnected=off
  AI_trigger_7_8 : Outport  Port=20  VectorParamsAs1DForOutWhenUnconnected=off
  AI_trigger_9_10 : Outport  Port=21  VectorParamsAs1DForOutWhenUnconnected=off
  AI_trigger_11_12 : Outport  Port=22  VectorParamsAs1DForOutWhenUnconnected=off
  AI_trigger_13_14 : Outport  Port=23  VectorParamsAs1DForOutWhenUnconnected=off
  AI_trigger_15_16 : Outport  Port=24  VectorParamsAs1DForOutWhenUnconnected=off
  AO_trigger_1_8 : Outport  Port=25  VectorParamsAs1DForOutWhenUnconnected=off
  AO_trigger_9_16 : Outport  Port=26  VectorParamsAs1DForOutWhenUnconnected=off
  cpu_AI : Outport  Port=27  VectorParamsAs1DForOutWhenUnconnected=off
  wires:
  IO3xx PCI Read/1 -> UnPacker/1(packed)
  UnPacker/1(unpacked) -> cpu_AI/1
  ground25/1 -> AO_trigger_9_16/1
  ground24/1 -> AO_trigger_1_8/1
  ground23/1 -> AI_trigger_15_16/1
  ground22/1 -> AI_trigger_13_14/1
  ground21/1 -> AI_trigger_11_12/1
  ground20/1 -> AI_trigger_9_10/1
  ground19/1 -> AI_trigger_7_8/1
  ground18/1 -> AI_trigger_5_6/1
  ground17/1 -> AI_trigger_3_4/1
  ground16/1 -> AI_trigger_1_2/1
  ground15/1 -> AO16/1
  ground14/1 -> AO15/1
  ground13/1 -> AO14/1
  ground12/1 -> AO13/1
  ground11/1 -> AO12/1
  ground10/1 -> AO11/1
  ground9/1 -> AO10/1
  ground8/1 -> AO9/1
  ground7/1 -> AO8/1
  ground6/1 -> AO7/1
  ground5/1 -> AO6/1
  ground4/1 -> AO5/1
  ground3/1 -> AO4/1
  ground2/1 -> AO3/1
  ground1/1 -> AO2/1
  ground/1 -> AO1/1
  Packer/1(packed) -> IO3xx PCI Write/1
  cpu_AO/1 -> Packer/1(unpacked)
  AI_valid_15_16/1 -> terminator23/1
  AI_valid_13_14/1 -> terminator22/1
  AI_valid_11_12/1 -> terminator21/1
  AI_valid_9_10/1 -> terminator20/1
  AI_valid_7_8/1 -> terminator19/1
  AI_valid_5_6/1 -> terminator18/1
  AI_valid_3_4/1 -> terminator17/1
  AI_valid_1_2/1 -> terminator16/1
  AI16/1 -> terminator15/1
  AI15/1 -> terminator14/1
  AI14/1 -> terminator13/1
  AI13/1 -> terminator12/1
  AI12/1 -> terminator11/1
  AI11/1 -> terminator10/1
  AI10/1 -> terminator9/1
  AI9/1 -> terminator8/1
  AI8/1 -> terminator7/1
  AI7/1 -> terminator6/1
  AI6/1 -> terminator5/1
  AI5/1 -> terminator4/1
  AI4/1 -> terminator3/1
  AI3/1 -> terminator2/1
  AI2/1 -> terminator1/1
  AI1/1 -> terminator/1

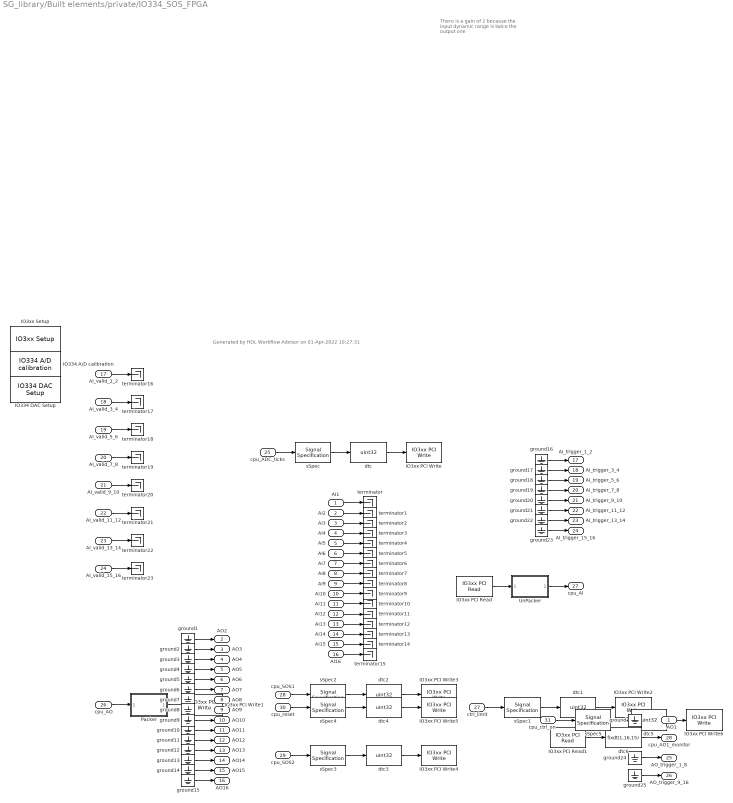
== system SG_library/Built elements/private/IO334_SOS_FPGA ==
  note: Generated by HDL Workflow Advisor on 01-Apr-2022 10:27:31
  note: There is a gain of 2 because the input dynamic range is twice the output one
  AI1 : Inport
  AI2 : Inport  Port=2
  AI3 : Inport  Port=3
  AI4 : Inport  Port=4
  AI5 : Inport  Port=5
  AI6 : Inport  Port=6
  AI7 : Inport  Port=7
  AI8 : Inport  Port=8
  AI9 : Inport  Port=9
  AI10 : Inport  Port=10
  AI11 : Inport  Port=11
  AI12 : Inport  Port=12
  AI13 : Inport  Port=13
  AI14 : Inport  Port=14
  AI15 : Inport  Port=15
  AI16 : Inport  Port=16
  AI_valid_1_2 : Inport  Port=17
  AI_valid_3_4 : Inport  Port=18
  AI_valid_5_6 : Inport  Port=19
  AI_valid_7_8 : Inport  Port=20
  AI_valid_9_10 : Inport  Port=21
  AI_valid_11_12 : Inport  Port=22
  AI_valid_13_14 : Inport  Port=23
  AI_valid_15_16 : Inport  Port=24
  cpu_ADC_ticks : Inport  Port=25
  cpu_AO : Inport  Port=26
  ctrl_limit : Inport  Port=27
  cpu_SOS1 : Inport  Port=28
  cpu_SOS2 : Inport  Port=29
  cpu_reset : Inport  Port=30
  cpu_ctrl_on : Inport  Port=31
  IO334 A/D calibration : speedgoatlib_hdlCoder_IO3xx/IO334 A//D calibration  module_id=module_id
  IO334 DAC Setup : speedgoatlib_hdlCoder_IO3xx/IO334 DAC Setup  module_id=module_id  OutputRange=Auto (same as ADC)
  IO3xx PCI Read : speedgoatlib_hdlCoder_IO3xx/IO3xx PCI Read  device_id=deviceIdx  module_id=module_id  board_type=IO3xx  port_name=cpu_AI  port_offset=hex2dec('220')  port_type=uint32  port_dim=8  strobe=hex2dec('240')  sample_time=ts
  IO3xx PCI Read1 : speedgoatlib_hdlCoder_IO3xx/IO3xx PCI Read  device_id=deviceIdx  module_id=module_id  board_type=IO3xx  port_name=cpu_AO1_monitor  port_offset=hex2dec('110')  port_type=uint32  port_dim=1  strobe=0  sample_time=ts
  IO3xx PCI Write : speedgoatlib_hdlCoder_IO3xx/IO3xx PCI Write  device_id=deviceIdx  module_id=module_id  board_type=IO3xx  port_name=cpu_ADC_ticks  port_offset=hex2dec('100')  port_type=uint32  port_dim=1  strobe=0  sample_time=ts
  IO3xx PCI Write1 : speedgoatlib_hdlCoder_IO3xx/IO3xx PCI Write  device_id=deviceIdx  module_id=module_id  board_type=IO3xx  port_name=cpu_AO  port_offset=hex2dec('120')  port_type=uint32  port_dim=8  strobe=hex2dec('140')  sample_time=ts
  IO3xx PCI Write2 : speedgoatlib_hdlCoder_IO3xx/IO3xx PCI Write  device_id=deviceIdx  module_id=module_id  board_type=IO3xx  port_name=ctrl_limit  port_offset=hex2dec('104')  port_type=uint32  port_dim=1  strobe=0  sample_time=ts
  IO3xx PCI Write3 : speedgoatlib_hdlCoder_IO3xx/IO3xx PCI Write  device_id=deviceIdx  module_id=module_id  board_type=IO3xx  port_name=cpu_SOS1  port_offset=hex2dec('180')  port_type=uint32  port_dim=24  strobe=hex2dec('200')  sample_time=ts
  IO3xx PCI Write4 : speedgoatlib_hdlCoder_IO3xx/IO3xx PCI Write  device_id=deviceIdx  module_id=module_id  board_type=IO3xx  port_name=cpu_SOS2  port_offset=hex2dec('280')  port_type=uint32  port_dim=24  strobe=hex2dec('300')  sample_time=ts
  IO3xx PCI Write5 : speedgoatlib_hdlCoder_IO3xx/IO3xx PCI Write  device_id=deviceIdx  module_id=module_id  board_type=IO3xx  port_name=cpu_reset  port_offset=hex2dec('108')  port_type=uint32  port_dim=1  strobe=0  sample_time=ts
  IO3xx PCI Write6 : speedgoatlib_hdlCoder_IO3xx/IO3xx PCI Write  device_id=deviceIdx  module_id=module_id  board_type=IO3xx  port_name=cpu_ctrl_on  port_offset=hex2dec('10C')  port_type=uint32  port_dim=1  strobe=0  sample_time=ts
  IO3xx Setup : speedgoatlib_hdlCoder_IO3xx/IO3xx Setup  mdl_ss_name=IO334_SOS_src/IO334_SOS_FPGA  board_type=IO334-325k  fpga_sync_mode=on  reset_mode=on  device_id=deviceIdx  module_id=module_id  pci_slot=slot  fpga_mat_file=C:\Speedgoat\Build\IO334_SOS\hdlsrc\IO334_SOS_src\IO334_SOS_FPGA.mat  timestamp_mcs=03/18/22 18:06:29  timestamp=2203181708  tsreg=hex2dec('8')  bsf_file=IO334_SOS_FPGA_2203181708.mcs  mcs=0
  Packer : Subsystem
  UnPacker : Subsystem
  dtc{,1..5} (6 alike) : DataTypeConversion  OutDataTypeStr=uint32  ConvertRealWorld=Stored Integer (SI)  RndMeth=Zero
  dtc6 : DataTypeConversion  OutDataTypeStr=fixdt(1,16,15)  ConvertRealWorld=Stored Integer (SI)  RndMeth=Zero
  ground{,1..25} (26 alike) : Ground
  sSpec : SignalSpecification  OutDataTypeStr=fixdt(0,32,0)
  sSpec1 : SignalSpecification  OutDataTypeStr=fixdt(1,16,15)
  sSpec2 : SignalSpecification  OutDataTypeStr=fixdt(1,32,20)
  sSpec3 : SignalSpecification  OutDataTypeStr=fixdt(1,32,20)
  sSpec4 : SignalSpecification  OutDataTypeStr=fixdt('boolean')
  sSpec5 : SignalSpecification  OutDataTypeStr=fixdt('boolean')
  terminator{,1..23} (24 alike) : Terminator
  AO1 : Outport  VectorParamsAs1DForOutWhenUnconnected=off
  AO2 : Outport  Port=2  VectorParamsAs1DForOutWhenUnconnected=off
  AO3 : Outport  Port=3  VectorParamsAs1DForOutWhenUnconnected=off
  AO4 : Outport  Port=4  VectorParamsAs1DForOutWhenUnconnected=off
  AO5 : Outport  Port=5  VectorParamsAs1DForOutWhenUnconnected=off
  AO6 : Outport  Port=6  VectorParamsAs1DForOutWhenUnconnected=off
  AO7 : Outport  Port=7  VectorParamsAs1DForOutWhenUnconnected=off
  AO8 : Outport  Port=8  VectorParamsAs1DForOutWhenUnconnected=off
  AO9 : Outport  Port=9  VectorParamsAs1DForOutWhenUnconnected=off
  AO10 : Outport  Port=10  VectorParamsAs1DForOutWhenUnconnected=off
  AO11 : Outport  Port=11  VectorParamsAs1DForOutWhenUnconnected=off
  AO12 : Outport  Port=12  VectorParamsAs1DForOutWhenUnconnected=off
  AO13 : Outport  Port=13  VectorParamsAs1DForOutWhenUnconnected=off
  AO14 : Outport  Port=14  VectorParamsAs1DForOutWhenUnconnected=off
  AO15 : Outport  Port=15  VectorParamsAs1DForOutWhenUnconnected=off
  AO16 : Outport  Port=16  VectorParamsAs1DForOutWhenUnconnected=off
  AI_trigger_1_2 : Outport  Port=17  VectorParamsAs1DForOutWhenUnconnected=off
  AI_trigger_3_4 : Outport  Port=18  VectorParamsAs1DForOutWhenUnconnected=off
  AI_trigger_5_6 : Outport  Port=19  VectorParamsAs1DForOutWhenUnconnected=off
  AI_trigger_7_8 : Outport  Port=20  VectorParamsAs1DForOutWhenUnconnected=off
  AI_trigger_9_10 : Outport  Port=21  VectorParamsAs1DForOutWhenUnconnected=off
  AI_trigger_11_12 : Outport  Port=22  VectorParamsAs1DForOutWhenUnconnected=off
  AI_trigger_13_14 : Outport  Port=23  VectorParamsAs1DForOutWhenUnconnected=off
  AI_trigger_15_16 : Outport  Port=24  VectorParamsAs1DForOutWhenUnconnected=off
  AO_trigger_1_8 : Outport  Port=25  VectorParamsAs1DForOutWhenUnconnected=off
  AO_trigger_9_16 : Outport  Port=26  VectorParamsAs1DForOutWhenUnconnected=off
  cpu_AI : Outport  Port=27  VectorParamsAs1DForOutWhenUnconnected=off
  cpu_AO1_monitor : Outport  Port=28  VectorParamsAs1DForOutWhenUnconnected=off
  wires:
  IO3xx PCI Read1/1 -> dtc6/1
  dtc6/1 -> cpu_AO1_monitor/1
  IO3xx PCI Read/1 -> UnPacker/1(packed)
  UnPacker/1(unpacked) -> cpu_AI/1
  ground25/1 -> AO_trigger_9_16/1
  ground24/1 -> AO_trigger_1_8/1
  ground23/1 -> AI_trigger_15_16/1
  ground22/1 -> AI_trigger_13_14/1
  ground21/1 -> AI_trigger_11_12/1
  ground20/1 -> AI_trigger_9_10/1
  ground19/1 -> AI_trigger_7_8/1
  ground18/1 -> AI_trigger_5_6/1
  ground17/1 -> AI_trigger_3_4/1
  ground16/1 -> AI_trigger_1_2/1
  ground15/1 -> AO16/1
  ground14/1 -> AO15/1
  ground13/1 -> AO14/1
  ground12/1 -> AO13/1
  ground11/1 -> AO12/1
  ground10/1 -> AO11/1
  ground9/1 -> AO10/1
  ground8/1 -> AO9/1
  ground7/1 -> AO8/1
  ground6/1 -> AO7/1
  ground5/1 -> AO6/1
  ground4/1 -> AO5/1
  ground3/1 -> AO4/1
  ground2/1 -> AO3/1
  ground1/1 -> AO2/1
  ground/1 -> AO1/1
  dtc5/1 -> IO3xx PCI Write6/1
  sSpec5/1 -> dtc5/1
  cpu_ctrl_on/1 -> sSpec5/1
  dtc4/1 -> IO3xx PCI Write5/1
  sSpec4/1 -> dtc4/1
  cpu_reset/1 -> sSpec4/1
  dtc3/1 -> IO3xx PCI Write4/1
  sSpec3/1 -> dtc3/1
  cpu_SOS2/1 -> sSpec3/1
  dtc2/1 -> IO3xx PCI Write3/1
  sSpec2/1 -> dtc2/1
  cpu_SOS1/1 -> sSpec2/1
  dtc1/1 -> IO3xx PCI Write2/1
  sSpec1/1 -> dtc1/1
  ctrl_limit/1 -> sSpec1/1
  Packer/1(packed) -> IO3xx PCI Write1/1
  cpu_AO/1 -> Packer/1(unpacked)
  dtc/1 -> IO3xx PCI Write/1
  sSpec/1 -> dtc/1
  cpu_ADC_ticks/1 -> sSpec/1
  AI_valid_15_16/1 -> terminator23/1
  AI_valid_13_14/1 -> terminator22/1
  AI_valid_11_12/1 -> terminator21/1
  AI_valid_9_10/1 -> terminator20/1
  AI_valid_7_8/1 -> terminator19/1
  AI_valid_5_6/1 -> terminator18/1
  AI_valid_3_4/1 -> terminator17/1
  AI_valid_1_2/1 -> terminator16/1
  AI16/1 -> terminator15/1
  AI15/1 -> terminator14/1
  AI14/1 -> terminator13/1
  AI13/1 -> terminator12/1
  AI12/1 -> terminator11/1
  AI11/1 -> terminator10/1
  AI10/1 -> terminator9/1
  AI9/1 -> terminator8/1
  AI8/1 -> terminator7/1
  AI7/1 -> terminator6/1
  AI6/1 -> terminator5/1
  AI5/1 -> terminator4/1
  AI4/1 -> terminator3/1
  AI3/1 -> terminator2/1
  AI2/1 -> terminator1/1
  AI1/1 -> terminator/1
